simulink model "sistema_controlado"  (R2021a)
settings: Solver=VariableStepAuto  StartTime=0.0  StopTime=100  RelTol=1e-3
model workspace (MAT data in the model file):
  y0 = 3.14259265359
values from neighbouring files (symbols this model uses):
  x0 = x_next    [P3.m]    (also in P3_old.m = [0; 0; pi+0.01;0]; control_cart.m = x_control(:,k+1))
libraries: simulink x1
settings Model: Creator=marti  LastModifiedBy=sebag

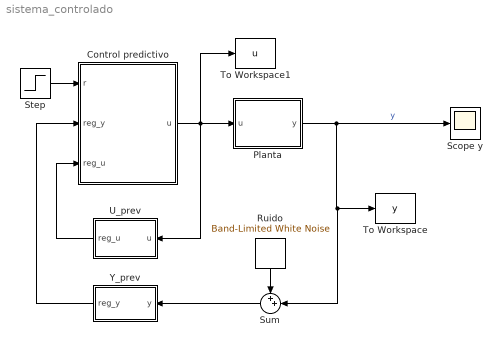
== system sistema_controlado ==
  Control predictivo : MATLAB Function  TreatAsAtomicUnit=on
  Planta : Subsystem
  Ruido : simulink/Sources/Band-Limited White Noise  Cov=[0.1]  Ts=0.1  seed=[23341]
  Scope y : Scope
  Step : Step  SampleTime=0
  Sum : Sum  Inputs=++|
  To Workspace : ToWorkspace  VariableName=y  SampleTime=-1
  To Workspace1 : ToWorkspace  VariableName=u  SampleTime=-1
  U_prev : Subsystem
  Y_prev : Subsystem
  wires:
  Control predictivo/1(u) -> To Workspace1/1, U_prev/1(u), Planta/1(u)
  Planta/1(y) -> Scope y/1, Sum/2, To Workspace/1  "y"
  Y_prev/1(reg_y) -> Control predictivo/2(reg_y)
  U_prev/1(reg_u) -> Control predictivo/3(reg_u)
  Step/1 -> Control predictivo/1(r)
  Sum/1 -> Y_prev/1(y)
  Ruido/1 -> Sum/1

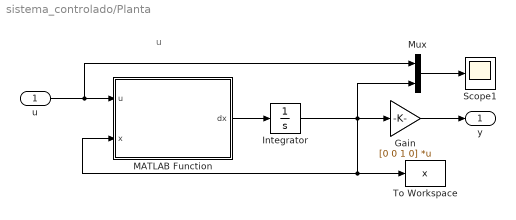
== system sistema_controlado/Planta ==
  note: u
  u : Inport
  Gain : Gain  Gain=[0 0 1 0]  Multiplication=Matrix(K*u)
  Integrator : Integrator  InitialCondition=x0
  MATLAB Function : MATLAB Function  TreatAsAtomicUnit=on
  Mux : Mux  Inputs=2
  Scope1 : Scope
  To Workspace : ToWorkspace  VariableName=x  SampleTime=-1
  y : Outport
  wires:
  MATLAB Function/1(dx) -> Integrator/1
  u/1 -> Mux/1, MATLAB Function/1(u)
  Integrator/1 -> Mux/2, Gain/1, To Workspace/1, MATLAB Function/2(x)
  Mux/1 -> Scope1/1
  Gain/1 -> y/1

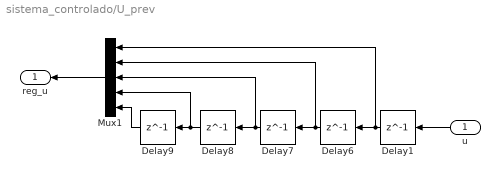
== system sistema_controlado/U_prev ==
  u : Inport
  Delay{1,6..9} (5 alike) : Delay  DelayLength=1
  Mux1 : Mux  Inputs=5
  reg_u : Outport
  wires:
  u/1 -> Delay1/1
  Delay8/1 -> Mux1/4, Delay9/1
  Delay6/1 -> Mux1/2, Delay7/1
  Delay7/1 -> Mux1/3, Delay8/1
  Delay9/1 -> Mux1/5
  Mux1/1 -> reg_u/1
  Delay1/1 -> Mux1/1, Delay6/1

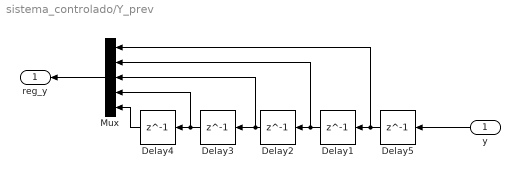
== system sistema_controlado/Y_prev ==
  y : Inport
  Delay{1..5} (5 alike) : Delay  DelayLength=1
  Mux : Mux  Inputs=5
  reg_y : Outport
  wires:
  Mux/1 -> reg_y/1
  y/1 -> Delay5/1
  Delay3/1 -> Mux/4, Delay4/1
  Delay2/1 -> Mux/3, Delay3/1
  Delay1/1 -> Mux/2, Delay2/1
  Delay4/1 -> Mux/5
  Delay5/1 -> Mux/1, Delay1/1

== matlab function sistema_controlado/Planta/MATLAB Function ==
  data: u input; x input; dx output
function dx = pendcart(u,x)
%x=[x,dx,theta,dtheta]
m = 1;
M = 5;
L = 2;
g = -9.8;
d = 1;

Sx = sin(x(3));
Cx = cos(x(3));
D = L*(M+m*(1-Cx^2));

dx=[x(2);(1/D)*(-m*L*g*Cx*Sx + L*(m*L*x(4)^2*Sx - d*x(2)) + L*u);...
    x(4);(1/D)*((m+M)*g*Sx - Cx*(m*L*x(4)^2*Sx - d*x(2)) - Cx*u)];
end

== matlab function sistema_controlado/Control predictivo ==
  data: r input; u output; reg_y input; reg_u input
function u = control(r,reg_y, reg_u)
coder.extrinsic('control_cart')
% Inducir el tamaño de los datos
yp = zeros(5,1);
up = zeros(5,1);
u = zeros(1,1);
r = r+1;
% Obtener los datos reales
yp = yp + reg_y;
up = up + reg_u;
% u = controller(yp, r, L, up, g, a, b);
u = 0;
end
